simulink model "Rearranged_With_Subsystems"  (R2022b)
settings: Solver=ode15s  StartTime=0.0  StopTime=400  RelTol=1e-3
InitFcn:
  | ManipulatorSetup
  | init_quad_new_leg_raibert_strategy_v2
values from neighbouring files (symbols this model uses):
  body = 'obstacle'+string(i)    [GUIWithNavigation.m]    (also in RunModel.m)
  endx = 18    [EnvironmentData.mat]    (also in Practice data.mat = 15)
  endy = 18    [EnvironmentData.mat]    (also in Practice data.mat = 14)
  floorl = 20    [EnvironmentData.mat]    (also in GUIWithNavigation.m; Practice data.mat; RunModel.m)
  floorw = 20    [EnvironmentData.mat]    (also in GUIWithNavigation.m; Practice data.mat; RunModel.m)
  planner = plannerRRTStar(ss,stateValidator)    [GUIWithNavigation.m]    (also in RunModel.m)
  startx = 3    [EnvironmentData.mat]    (also in Practice data.mat = 2)
  starty = 3    [EnvironmentData.mat]    (also in Practice data.mat = 2)
  tar1Len = 10    [EnvironmentData.mat]    (also in GUIWithNavigation.m = length(target1); Practice data.mat = 13; RunModel.m = length(target1))
  target = [3 4.99844642156 6.95141646815 8.78790598722 9.67257563911 9.70990834754 10.5092252376 9.30187214417 9.05327436398 9.4 9.4 10.8486938703 ... (44 elements, 22x2)]    [EnvironmentData.mat]    (also in GUIWithNavigation.m = cat(1,target1,target2); Practice data.mat = [2 3.44057581018 5.07942513831 5.42542290116 7.21306818311 8; RunModel.m = cat(1,target1,target2))
  tarLen = 22    [EnvironmentData.mat]    (also in RunModel.m = length(target))
undefined symbols (not defined in the file or in its folder): closeFingers, ctrl, Extr_Data_LinkEndHole, grabObjectAngles, grabObjectAngles2, ground, holdFingers, homeAngles, inverseKinematicWeights, l1, l2, m1, m2, openFingers, readyAngles, X, Y, Z
libraries: sm_lib x459, nesl_utility x134, slpidlib x31, fl_ps_legacy_lib x6, robotmaniplib x6, simulink x5, fl_lib x5, Contact_Forces_Lib x4, Parts_Lib x4, sharedtransform x2, dspstat3 x1
(part 16 of 16)

== matlab function Rearranged_With_Subsystems/Manipulator/MATLAB Function ==
  settings: updateMethod=DISCRETE
  data: quadrupedInPosition input; errorVals input; state input; readyAngles input; openFingers input; closeFingers input; objectPosition input; aboveObjectPosition input; endPos input; aboveEndPos input; time input; y output; stateOut output; getBallPos output; getEndPos output; ballGot output
function [y,stateOut,getBallPos,getEndPos,ballGot] = fcn(quadrupedInPosition,errorVals,state,readyAngles,openFingers,closeFingers,objectPosition,aboveObjectPosition,endPos,aboveEndPos,time)

persistent startTime
if isempty(startTime)
    startTime=0;
end

threshold=0.05;
if quadrupedInPosition == 1
    state = int16(state);

    switch state
        case 0
            y = [readyAngles;openFingers];
            getBallPos=0;
            getEndPos=0;
            ballGot=0;
        case 1
            getBallPos=0;
            getEndPos=0;
            y = [aboveObjectPosition;openFingers];
            ballGot=0;
        case 2
            getBallPos=0;
            getEndPos=0;
            y = [objectPosition;openFingers];
            ballGot=0;
        case 3
            getBallPos=0;
            getEndPos=0;
            y = [objectPosition;closeFingers];
            ballGot=0;
        case 4
            getBallPos=0;
            getEndPos=0;
            y = [aboveObjectPosition;closeFingers];
            ballGot=1;
        case 5
            getBallPos=0;
            getEndPos=0;
            y = [readyAngles;closeFingers];
            ballGot=1;
        otherwise
            y = zeros(13,1);
            getBallPos=0;
            getEndPos=0;
            ballGot=0;
    end
    
    if state == 0 && min(errorVals) >= -threshold && max(errorVals) <=threshold
        getBallPos=1;
        stateOut = 1;
        startTime=time;
    elseif state == 1 && min(errorVals) >= -threshold && max(errorVals) <=threshold && (time-startTime) >= 4
        getBallPos=1;
        stateOut = 2;
        startTime=time;
    elseif state == 2  && (time-startTime) >= 4
        stateOut = 3;
        startTime=time;
    elseif state==3 && min(errorVals) >= -threshold && max(errorVals) <=threshold && (time-startTime) >= 4
        stateOut = 4;
        startTime=time;
    elseif state == 4 && min(errorVals) >= -threshold && max(errorVals) <=threshold && (time-startTime) >= 4
        stateOut = 5;
        startTime=time;
    elseif state == 5 && min(errorVals) >= -threshold && max(errorVals) <=threshold && (time-startTime)>=4
        stateOut = 5;
    else
        stateOut = double(state);
    end

elseif quadrupedInPosition == 2

    switch state
        case 5
            y = [readyAngles;closeFingers];
            getBallPos=0;
            getEndPos=0;
            ballGot=1;
        case 6
            getBallPos=0;
            getEndPos=0;
            y = [aboveEndPos;closeFingers];
            ballGot=1;
        case 7
            getBallPos=0;
            getEndPos=0;
            y = [endPos;closeFingers];
            ballGot=1;
        case 8
            getBallPos=0;
            getEndPos=0;
            y = [endPos;openFingers];
            ballGot=1;
        case 9
            getBallPos=0;
            getEndPos=0;
            y = [aboveEndPos;openFingers];
            ballGot=0;
        case 10
            getBallPos=0;
            getEndPos=0;
            y = [readyAngles;openFingers];
            ballGot=0;
        case 11
            getBallPos=0;
            getEndPos=0;
            y = [readyAngles;openFingers];
            ballGot=0;
        otherwise
            y = zeros(13,1);
            getBallPos=0;
            getEndPos=0;
            ballGot=0;
    end
    if state == 5 && min(errorVals) >= -threshold && max(errorVals) <=threshold
        stateOut = 6;
        startTime=time;
    elseif state == 6 && min(errorVals) >= -threshold && max(errorVals) <=threshold && (time-startTime) >= 4
        getEndPos=1;
        stateOut = 7;
        startTime=time;
    elseif state == 7  && (time-startTime) >= 4
        stateOut = 8;
        startTime=time;
    elseif state==8 && min(errorVals) >= -threshold && max(errorVals) <=threshold && (time-startTime) >= 5
        stateOut = 9;
        startTime=time;
    elseif state == 9 && min(errorVals) >= -threshold && max(errorVals) <=threshold && (time-startTime) >= 10
        stateOut = 10;
        startTime=time;
    elseif state == 10 && min(errorVals) >= -threshold && max(errorVals) <=threshold && (time-startTime)>=4
        stateOut = 11;
        startTime=time;
    elseif state == 11 && min(errorVals) >= -threshold && max(errorVals) <=threshold && (time-startTime)>=4
        stateOut = 11;
    else
        stateOut = double(state);
    end
else
    y = [readyAngles;openFingers];
    stateOut = 0;
    getBallPos=0;
    getEndPos=0;
    ballGot=0;
end

== matlab function Rearranged_With_Subsystems/Manipulator/Subsystem1/Manipulator interpolator ==
  settings: updateMethod=DISCRETE
  data: desiredAngles input size=[7  1]; angleRangeOut output size=[1 14]; currentAngles input size=[7 1]; timeRangeOut output size=[1 14]; time input; debug output
function [angleRangeOut,timeRangeOut,debug]  = manipInterp(desiredAngles,currentAngles,time)

persistent beginState
persistent ready1
persistent ready2
persistent ready3
persistent ready4
persistent ready5
persistent ready6
persistent ready7

% persistent interval
persistent startTime
persistent angleRange
persistent timeRange

if isempty(beginState)
    beginState=transpose(currentAngles);
end

% if isempty(interval)
%     interval=0.01;
% end
if isempty(startTime)
    startTime=10;
end
if isempty(angleRange)
    angleRange=[transpose(currentAngles),transpose(currentAngles)];
end
if isempty(timeRange)
    timeRange=[ones(1,7)*0,ones(1,7)*600];
end
if isempty(ready1)
    ready1=0;
end
if isempty(ready2)
    ready2=0;
end
if isempty(ready3)
    ready3=0;
end
if isempty(ready4)
    ready4=0;
end
if isempty(ready5)
    ready5=0;
end
if isempty(ready6)
    ready6=0;
end
if isempty(ready7)
    ready7=0;
end

%timeSteps=0.01;
transferTime=3;
%calcTime=timeSteps/transferTime;
angleDif=transpose(abs(desiredAngles-currentAngles));
threshold=0.01;
TcurrentAngles=transpose(currentAngles);
if angleDif(1)>=threshold||angleDif(2)>=threshold||angleDif(3)>=threshold||angleDif(4)>=threshold||angleDif(5)>=threshold||angleDif(6)>=threshold||angleDif(7)>=threshold
    if ready1==0&&ready2==0&&ready3==0&&ready4==0&&ready5==0&&ready6==0&&ready7==0
        beginState=transpose(currentAngles);
        %interval=((desiredAngles-beginState)./calcTime);
        startTime=time;
        ready1=1;
        ready2=1;
        ready3=1;
        ready4=1;
        ready5=1;
        ready6=1;
        ready7=1;
        endTime=transferTime+startTime;
        timeRange=[ones(1,7)*startTime,ones(1,7)*endTime];
        angleRange=[beginState,transpose(desiredAngles)];
    end       
end

if angleDif(1)<=threshold
    ready1=0;
    timeRange(1)=0;
    timeRange(8)=600;
    angleRange(1)=TcurrentAngles(1);
    angleRange(8)=TcurrentAngles(1);
end
if angleDif(2)<=threshold
    ready2=0;
    timeRange(2)=0;
    timeRange(9)=600;
    angleRange(2)=TcurrentAngles(2);
    angleRange(9)=TcurrentAngles(2);
end
if angleDif(3)<=threshold
    ready3=0;
    timeRange(3)=0;
    timeRange(10)=600;
    angleRange(3)=TcurrentAngles(3);
    angleRange(10)=TcurrentAngles(3);
end
if angleDif(4)<=threshold
    ready4=0;
    timeRange(4)=0;
    timeRange(11)=600;
    angleRange(4)=TcurrentAngles(4);
    angleRange(11)=TcurrentAngles(4);
end
if angleDif(5)<=threshold
    ready5=0;
    timeRange(5)=0;
    timeRange(12)=600;
    angleRange(5)=TcurrentAngles(5);
    angleRange(12)=TcurrentAngles(5);
end
if angleDif(6)<=threshold
    ready6=0;
    timeRange(6)=0;
    timeRange(13)=600;
    angleRange(6)=TcurrentAngles(6);
    angleRange(13)=TcurrentAngles(6);
end
if angleDif(7)<=threshold
    ready7=0;
    timeRange(7)=0;
    timeRange(14)=600;
    angleRange(7)=TcurrentAngles(7);
    angleRange(14)=TcurrentAngles(7);
end

angleRangeOut=angleRange;
timeRangeOut=timeRange;
debug=angleDif;

== matlab function Rearranged_With_Subsystems/Controller/MATLAB Function1 ==
  settings: updateMethod=DISCRETE
  data: go input; mode output; targets input; tar1Len input; tarLen input; x input; y input; angle input; done output
function [mode,done] = broadside(go,targets,tar1Len,tarLen,x,y,angle)

persistent targetAssigned
if isempty(targetAssigned)
    targetAssigned=0;
end

persistent broadTarget
if isempty(broadTarget)
    broadTarget=[0,0];
end

persistent points
if isempty(points)
    points=0;
end

persistent point1
if isempty(point1)
    point1=[0,0];
end

persistent point2
if isempty(point2)
    point2=[0,0];
end

persistent currentTarget
if isempty(currentTarget)
    currentTarget=[0,0];
end


if go==1||go==2
    if targetAssigned==0
        if go==1
            broadTarget=targets(tar1Len,:);
        elseif go==2
            broadTarget=targets(tarLen,:);
        end
        if y>broadTarget(2)
            spacing=1;
        else
            spacing=-1;
        end
        if x>broadTarget(1)
            points=2;
            point1=[x,broadTarget(2)+spacing];
            point2=[broadTarget(1),broadTarget(2)+spacing];
        else
            points=1;
            point1=[broadTarget(1),broadTarget(2)+spacing];
        end
        currentTarget=point1;
        targetAssigned=1;
    end
    delta=currentTarget-[x,y];
    deltaDist=sqrt(delta(1).^2+delta(2).^2);
    targetAngle=atan2(delta(2),delta(1));
    deltaAngle=targetAngle-angle;
    if abs(deltaDist)>=0.1
        if deltaAngle<-0.1
            %disp('im left')
            %turn right
            mode=2;

        elseif deltaAngle>0.1
            %disp('im right')
            %turn left
            mode=3;
        else
            %disp('im forward')
            mode=1;
        end
        done=0;
    else
        if (currentTarget-point1)*[1;1]==0&&points==1
            currentTarget=[broadTarget(1),broadTarget(2)];
            done=0;
        elseif (currentTarget-point1)*[1;1]==0&&points==2
            currentTarget=point2;
            done=0;
        elseif (currentTarget-point2)*[1;1]==0
            currentTarget=[broadTarget(1),broadTarget(2)];
            done=0;
        else
            done=1;
        end
        mode=0;
    end
else
    targetAssigned=0;
    done=0;
    mode=0;
end

== stateflow chart Rearranged_With_Subsystems/Controller/Subsystem/Chart ==
  state PathFollowing
    endSim=false;
    resetPos=0;
    sqrt((target(tar1Len,1)-x).^2+ (target(tar1Len,2)-y).^2)
  state ManipulatorTask1
    resetPos=1;
  state PathFollowing2
    resetPos=0;
    sqrt((target(tar1Len,1)-x).^2+ (target(tar1Len,2)-y).^2)
  state ManipulatorTask2
    resetPos=2;
  state EndSim
    resetPos=0;
    endSim=true;
  (default) -> PathFollowing
  PathFollowing -> ManipulatorTask1 : [sqrt((target(tar1Len,1)-x).^2+ (target(tar1Len,2)-y).^2)<=1]{posToSkip=tar1Len-pos_index}
  ManipulatorTask1 -> PathFollowing2 : [manipState>=5]
  PathFollowing2 -> ManipulatorTask2 : [sqrt((target(tarLen,1)-x).^2+ (target(tarLen,2)-y).^2)<=1]
  ManipulatorTask2 -> EndSim : [manipState>=11]
  data: tar1Len input; resetPos output; manipState input; tarLen input; targetReached input; endSim output; check input; target input; y input; posToSkip output; x input; pos_index input

== stateflow chart Rearranged_With_Subsystems/Controller/High Level Mode Stateflow2 ==
  state ManipTask1
    ManipTask=1;
  state Broadside
    broadside=1;
  note: 0.35
  note: 1
  state ResetPos1
    mode=0;
  state Stationary
    mode=0;
  state Turning_Left
    mode=3;
  state Turning_Right
    mode=2;
  state Walking
    mode=1;
  state ResetPos2
    mode=0;
  state Broadside1
    broadside=2;
  state ManipTask2
    ManipTask=2;
  ManipTask1 -> Stationary : [resetPos==0]
  Broadside -> ManipTask1 : [broadFinished==1&&stopped]{broadside=0}
  ResetPos1 -> Broadside : [stopped]{pos_index=pos_index+1+posToSkip}
  Turning_Right -> ResetPos1 [order 2] : [resetPos==1]
  Stationary -> ResetPos1 [order 2] : [resetPos==1]
  Walking -> ResetPos1 [order 5] : [resetPos==1]
  Turning_Left -> ResetPos1 [order 3] : [resetPos==1]
  Stationary -> Stationary [order 3] : [target_reached&&pos_index~=tarLen]
      | {pos_index = pos_index + 1}
  (default) -> Stationary : {pos_index =2;bodyMode=0}
  Turning_Left -> Stationary [order 1] : [delta_theta < ang_threshold]
  Turning_Right -> Stationary [order 1] : [delta_theta > -ang_threshold]
  Walking -> Stationary [order 3] : [target_reached&&pos_index~=tarLen]
      | {pos_index = pos_index + 1}
  Stationary -> ResetPos2 [order 4] : [resetPos==2]
  Stationary -> Walking [order 1] : [~target_reached]
  Walking -> Turning_Left [order 1] : [delta_theta > ang_threshold]
  Walking -> Turning_Right [order 2] : [delta_theta < -ang_threshold]
  Turning_Left -> ResetPos2 [order 2] : [resetPos==2]
  Turning_Right -> ResetPos2 [order 3] : [resetPos==2]
  Walking -> ResetPos2 [order 4] : [resetPos==2]
  ResetPos2 -> Broadside1 : [stopped]
  Broadside1 -> ManipTask2 : [broadFinished==1&&stopped]{broadside=0}
  data: pos_index output =0; mode output =0; target_reached input; delta_theta input; ang_threshold local =0.2; resetPos input; ManipTask output; stopped input; bodyMode output; tarLen input; broadside output; broadFinished input; posToSkip input

== stateflow chart Rearranged_With_Subsystems/Controller/State Transitions ==
  state Initilisation
    next_state = 1;
  state Walking_Phase_fr_rl
    next_state = 2;
  state Stationary
    next_state = 4;
  state Walking_Phase_fl_rr
    next_state = 3;
  (default) -> Initilisation
  Initilisation -> Stationary : [ctrl_state==next_state]
  Stationary -> Walking_Phase_fr_rl : [mode >= 1 && ctrl_state == next_state]
  Walking_Phase_fl_rr -> Walking_Phase_fr_rl [order 2] : [ctrl_state == next_state]
  Walking_Phase_fr_rl -> (junction 49) [order 1] : [mode == 0]
  Walking_Phase_fr_rl -> Walking_Phase_fl_rr [order 2] : [ctrl_state == next_state]
  (junction 49) -> Stationary
  Walking_Phase_fl_rr -> (junction 49) [order 1] : [mode == 0]
  data: ctrl_state input =0; mode input =0; next_state output
